simulink subsystem "Plataforma_IGBT"  (R2024b)
settings: Solver=VariableStepAuto  StartTime=0.0  StopTime=10.0  RelTol=1e-3
values from neighbouring files (symbols this model uses):
  R_L = mean(RL)    [backup_0907.m]    (also in controller_0107.m = 0.01; matlabfunction_0207_ukf.m = 0.1)
  Ts = 0.001    [boost_data.mat]    (also in teste_ukf.m = 1e-05; wynda_demo.m)
undefined symbols (not defined in the file or in its folder): f_cutoff, var_HV, var_LV
libraries: fl_lib x18, ee_lib x18, nesl_utility x15
settings Model: Creator=eric  LastModifiedBy=eric

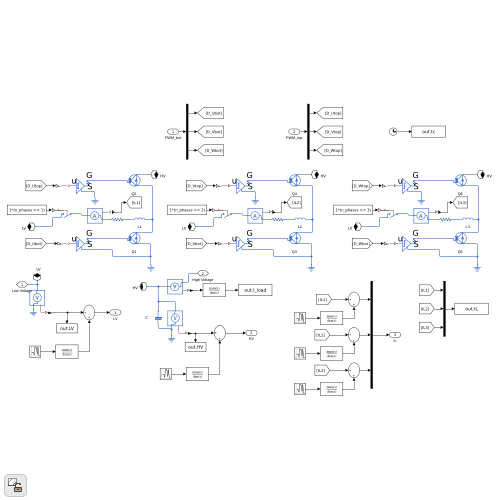
[thumbnail: Simulink's stored preview of the top-level diagram]
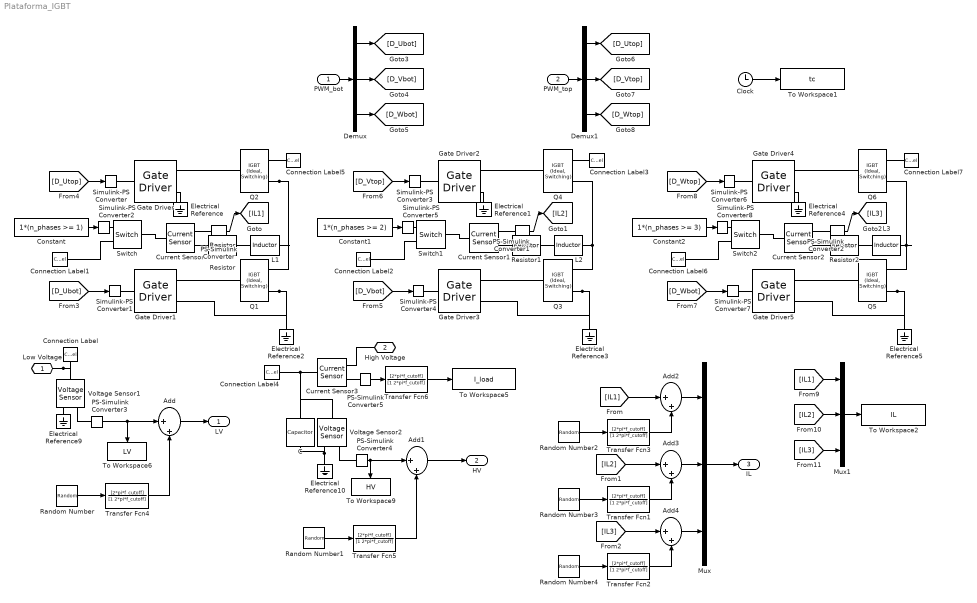
== system Plataforma_IGBT ==
  PWM_bot : Inport
  PWM_top : Inport  Port=2
  Add{,1..4} (5 alike) : Sum  Inputs=|++
  C : fl_lib/Electrical/Electrical Elements/Capacitor  c=C_out mF  r=C_out_esr mOhm  g=0 1/Ohm  i_specify=off  i_priority=None  i=0 A  i_nominal_specify=off  i_nominal_value=1  i_nominal_unit=A  v_specify=on  v_priority=None  v=12 V  v_nominal_specify=off  v_nominal_value=1  v_nominal_unit=V  vc_specify=off  vc_priority=High  vc=0 V  vc_nominal_specify=off  vc_nominal_value=1  vc_nominal_unit=V
  Clock : Clock
      settings: Decimation=decim
  Connection Label{,1..2,6} (4 alike) : ConnectionLabel  Label=LV
  Connection Label{3..5,7} (4 alike) : ConnectionLabel  Label=HV
  Constant : Constant  Value=1*(n_phases >= 1)
  Constant1 : Constant  Value=1*(n_phases >= 2)
  Constant2 : Constant  Value=1*(n_phases >= 3)
  Current Sensor{,1..3} (4 alike) : fl_lib/Electrical/Electrical Sensors/Current Sensor
  Demux : Demux  Outputs=3
  Demux1 : Demux  Outputs=3
  Electrical Reference{,1..5,9..10} (8 alike) : fl_lib/Electrical/Electrical Elements/Electrical Reference
  Gate Driver{,1..5} (6 alike) : ee_lib/Semiconductors & Converters/Gate Driver  port_option=ee.enum.controlport.ps  uHigh=2.0 V  uLow=0.8 V  uHighValue=0.7  uLowValue=0.3  vHigh=15 V  vLow=0 V  tHigh=50 ns  tLow=50 ns  parameterization=ee.enum.semiconductors.gateDriverParam.outputImpedance  rHigh=2 Ohm  rLow=2 Ohm  tRise=20 ns  tFall=20 ns  cLoad=10 nF  t_fault=1 s  ZonTime_specify=off  ZonTime_priority=None  ZonTime=0 s  ZoffTime_specify=off  ZoffTime_priority=None  ZoffTime=0 s
      settings: InternalSimscapePortConfiguration="{\"Bottom\":[],\"Left\":[{\"id\":\"u\",\"label\":\"u\",\"type\":\"input\"}],\"Right\":[{\"id\":\"G\",\"label\":\"G\",\"type\":\"foundation.electrical.electrical\"},{\"id\":\"S\",\"label\":\"S\",\"type\":\"foundation.electrical.electrical\"}],\"Top\":[]}"
  L1 : ee_lib/Passive/Inductor  l=L mH  enable_L_tol=ee.enum.toleranceApplication.applyRand  L_tol=10  tol_distribution=ee.enum.toleranceDistribution.uniform  nSigma=4  r=0 mOhm  g=1e-9 1/Ohm  enable_operating_limits=ee.enum.enable.no  operating_limit_action=ee.enum.passive.reportOpLim.warn  max_working_current=1 A  power_rating=1 W  fault_action=simscape.enum.assert.action.none  t_fault=1 s  i_L_specify=off  i_L_priority=High  i_L=0 A  i_L_nominal_specify=off  i_L_nominal_value=1  i_L_nominal_unit=A
  L2 : ee_lib/Passive/Inductor  l=L mH  enable_L_tol=ee.enum.toleranceApplication.applyRand  L_tol=10  tol_distribution=ee.enum.toleranceDistribution.uniform  nSigma=4  r=0 mOhm  g=1e-9 1/Ohm  enable_operating_limits=ee.enum.enable.no  operating_limit_action=ee.enum.passive.reportOpLim.warn  max_working_current=1 A  power_rating=1 W  fault_action=simscape.enum.assert.action.none  t_fault=1 s  i_L_specify=off  i_L_priority=High  i_L=0 A  i_L_nominal_specify=off  i_L_nominal_value=1  i_L_nominal_unit=A
  L3 : ee_lib/Passive/Inductor  l=L mH  enable_L_tol=ee.enum.toleranceApplication.applyRand  L_tol=10  tol_distribution=ee.enum.toleranceDistribution.uniform  nSigma=4  r=0 mOhm  g=1e-9 1/Ohm  enable_operating_limits=ee.enum.enable.no  operating_limit_action=ee.enum.passive.reportOpLim.warn  max_working_current=1 A  power_rating=1 W  fault_action=simscape.enum.assert.action.none  t_fault=1 s  i_L_specify=off  i_L_priority=High  i_L=0 A  i_L_nominal_specify=off  i_L_nominal_value=1  i_L_nominal_unit=A
  Mux : Mux  Inputs=3
  Mux1 : Mux  Inputs=3
  PS-Simulink Converter{,1..5} (6 alike) : nesl_utility/PS-Simulink Converter  PhysicalDomain=network_engine_domain  SubClassName=ps_output  LeftPortType=input  RightPortType=output  PseudoPeriodic=off  Frequencies=[]  VectorFormat=inherit  Unit=inherit  AffineConversion=off
  Q{1..6} (6 alike) : ee_lib/Semiconductors & Converters/IGBT (Ideal, Switching)  port_option=ee.enum.controlport.elec  Vf=0.8 V  Ron=0.001 Ohm  Goff=1e-5 1/Ohm  Vth=6 V  diode_param=ee.enum.semiconductors.protectionDiode.nodynamics  diode_Vf=0.8 V  diode_Ron=0.001 Ohm  diode_Goff=1e-5 1/Ohm  diode_C=50e-9 F  diode_iRM=-235 A  diode_iF=300 A  diode_idot=-50 A/us  diode_trr_param=ee.enum.converters.diodeReverseParam.trr_factor  diode_trr_factor=3  diode_trr=15 us  diode_Qrr=1500 s*uA  ice_specify=off  ice_priority=None  ice=0 A  ice_nominal_specify=off  ice_nominal_value=1  ice_nominal_unit=A  vce_specify=off  vce_priority=None  vce=0 V  vce_nominal_specify=off  vce_nominal_value=1  vce_nominal_unit=V  vge_specify=off  vge_priority=None  vge=0 V  vge_nominal_specify=off  vge_nominal_value=1  vge_nominal_unit=V  thermal_loss_option=ee.enum.converters.thermalLossOption.constantvalues  Von_data=[0, .1, .6, .8, 1, 1.3, 1.6, 2, 2.4; 0, .1, .7, 1, 1.2, 1.5, 1.9, 2.4, 2.8] V  Tj=[298.15, 398.15] K  Iout_data=[0, .1, 1, 5, 10, 20, 40, 70, 100] A  Eon_data=[0, .0024, .024, .12, .2, .48, 1.04, 2.16, 3.24; 0, .003, .03, .15, .25, .6, 1.3, 2.7, 4.05] * 1e-3 J  Eoff_data=[0, .0007, .0066, .033, .066, .17, .33, .83, 1.5; 0, .001, .01, .05, .1, .25, .5, 1.2, 2.2] * 1e-3 J  Eon_data_3D=[zeros(2, 9, 3)] J  Eoff_data_3D=[zeros(2, 9, 3)] J  Tj_loss=[298.15, 398.15] K  Iout_data_loss=[0, .1, 1, 5, 10, 20, 40, 70, 100] A  tabulateWithVce=false  Vce_loss=[0, 150, 300] V  Eon_scalar=22.86e-3 J  Eoff_scalar=17.14e-3 J  Voff=300 V  Iout_scalar=600 A  useCurrentFromPreviousCycle=false  useVoltageFromPreviousCycle=false  diodeModelType=ee.enum.converters.diodeModelType.pwl  diodeTableType=ee.enum.diode.tableType.IfMat  diode_ReverseIVType=ee.enum.diode.diodeReverseIV.constant  diode_IfMat=[.07, .12, .19, 1.75, 4.24, 7.32, 11.2; .16, .3, .72, 2.14, 4.02, 6.35, 9.12] A  diode_VfMat=[.9, 1.15, 1.25, 1.5, 1.75, 2.17, 2.6, 2.85; .58, .68, .75, 1.1, 1.38, 1.77, 2.27, 2.7] V  diode_TjVec=[25, 125] degC  diode_VfVec=[.5, .7, .9, 1.3, 1.7, 2.1, 2.5] V  diode_IfVec=[.1, .2, .5, 1, 2, 4, 7, 10] A  diode_IrMat=[1e-06, 2e-06, 5e-06, 1e-05, 2.5e-05, 5e-05, .0001; 2e-06, 5e-06, 1e-05, 4e-05, 8e-05, .0002, .0005] A  diode_VrMat=[10, 100, 200, 250, 300, 325, 350; 10, 70, 160, 220, 270, 300, 320] V  diode_VrVec=[10, 20, 40, 50, 70, 80, 100] V  diode_IrVec=[1e-06, 2e-06, 5e-06, 1e-05, 2e-05, 5e-05, .0001] A  diode_Vr=-600 V  diode_Ls=150 nH  diode_Erec=0.03 J  diode_rec_loss_model=ee.enum.diode.reverseRecoveryModel.fixed  diode_ErecVal=0 J  diode_scaleWithIandV=true  diode_ErecMat=zeros(2, 3) J  diode_TjrecVec=[298.15, 398.15] K  diode_IfrecVec=[.1, 1, 10] A  diode_IrecVal=10 A  diode_VrecVal=10 V  diode_tFilter=1 / 1000 / 100 s  separateThermalPortForDiode=false  thermal_network_parameterization=ee.enum.thermalNetworkTopology.external  Rth=[.08, .5] K/W  Rth_Cauer=[.08, .1, .5] K/W  Rth_Foster=[.08, .14, .22, .16] K/W  thermal_mass_parameterization=ee.enum.thermalNetwork.timeconstant  thermal_mass=[.01, .5] J/K  thermal_mass_Cauer=[.01, .1, .5] J/K  thermal_mass_Foster=[.001, .005, .05, .5] J/K  thermal_time_constant=[.001, .2] s  thermal_time_constant_Cauer=[.001, .1, .2] s  thermal_time_constant_Foster=[7e-05, .0007, .01, .08] s  thermal_mass_initial_temperatures=[25, 25] degC  thermal_mass_initial_temperatures_Cauer=[25, 25, 25] degC  junction_thermal_mass=0.01 J/K  Tvec_initial_Foster=[25, 25, 25, 25] degC  RthDiode=[.03, .2] K/W  RthCauerDiode=[.03, .1, .2] K/W  RthFosterDiode=[.03, .2] K/W  thermalMassDiode=[3, 25] J/K  thermalMassCauerDiode=[3, 10, 25] J/K  thermalMassFosterDiode=[33, 50] J/K  thermalTauDiode=[.1, 5] s  thermalTauCauerDiode=[.1, 1, 5] s  thermalTauFosterDiode=[1, 10] s  thermalMassInitTempDiode=[25, 25] degC  thermalMassInitTempCauerDiode=[25, 25, 25] degC  junctionthermalMassDiode=0.1 J/K  TVecInitialFosterDiode=[25, 25, 25, 25] degC  no_thermal_network=0  IGBT_junction_temperature_specify=off  IGBT_junction_temperature_priority=None  IGBT_junction_temperature=25 degC  IGBT_junction_temperature_nominal_specify=off  IGBT_junction_temperature_nominal_value=1  IGBT_junction_temperature_nominal_unit=degC  diode_junction_temperature_specify=off  diode_junction_temperature_priority=None  diode_junction_temperature=25 degC  diode_junction_temperature_nominal_specify=off  diode_junction_temperature_nominal_value=1  diode_junction_temperature_nominal_unit=degC  Qj_specify=off  Qj_priority=None  Qj=0 W  Qj_nominal_specify=off  Qj_nominal_value=1  Qj_nominal_unit=W  accumulatedSwitchingLosses_specify=off  accumulatedSwitchingLosses_priority=None  accumulatedSwitchingLosses=0 J
      settings: InternalSimscapePortConfiguration="{\"Bottom\":[],\"Left\":[{\"id\":\"G_elec\",\"label\":\"\",\"type\":\"foundation.electrical.electrical\"}],\"Right\":[{\"id\":\"C\",\"label\":\"\",\"type\":\"foundation.electrical.electrical\"},{\"id\":\"E\",\"label\":\"\",\"type\":\"foundation.electrical.electrical\"}],\"Top\":[]}"
  Random Number : RandomNumber  Variance=var_LV  SampleTime=Ts
  Random Number{1..4} (4 alike) : RandomNumber  Variance=var_HV  SampleTime=Ts
  Resistor : ee_lib/Passive/Resistor  R=R_L mOhm  enable_R_tol=ee.enum.toleranceApplication.applyRand  R_tol=50  tol_distribution=ee.enum.toleranceDistribution.uniform  nSigma=4  enable_operating_limits=ee.enum.enable.no  operating_limit_action=ee.enum.passive.reportOpLim.warn  power_rating=1 W  max_working_voltage=100 V  noise_mode=ee.enum.sources.noise.Disabled  Tdevice=25 degC  sample_time=1e-3 s  repeatability=ee.enum.ic.repeatability.notRepeatable  user_seed=0  auto_seed=3499211588  fault_action=simscape.enum.assert.action.none  t_fault=1 s  power_derating_T1=70 degC  power_derating_T2=155 degC  operating_temperature_range_vec=[-50, 150] degC  alpha=3.93e-3 1/K  Tmeas=25 degC  thermal_mass=100 J/K  temperature_specify=off  temperature_priority=High  temperature=298.15 K  temperature_nominal_specify=off  temperature_nominal_value=1  temperature_nominal_unit=K
  Resistor1 : ee_lib/Passive/Resistor  R=R_L mOhm  enable_R_tol=ee.enum.toleranceApplication.applyRand  R_tol=50  tol_distribution=ee.enum.toleranceDistribution.uniform  nSigma=4  enable_operating_limits=ee.enum.enable.no  operating_limit_action=ee.enum.passive.reportOpLim.warn  power_rating=1 W  max_working_voltage=100 V  noise_mode=ee.enum.sources.noise.Disabled  Tdevice=25 degC  sample_time=1e-3 s  repeatability=ee.enum.ic.repeatability.notRepeatable  user_seed=0  auto_seed=3890346746  fault_action=simscape.enum.assert.action.none  t_fault=1 s  power_derating_T1=70 degC  power_derating_T2=155 degC  operating_temperature_range_vec=[-50, 150] degC  alpha=3.93e-3 1/K  Tmeas=25 degC  thermal_mass=100 J/K  temperature_specify=off  temperature_priority=High  temperature=298.15 K  temperature_nominal_specify=off  temperature_nominal_value=1  temperature_nominal_unit=K
  Resistor2 : ee_lib/Passive/Resistor  R=R_L mOhm  enable_R_tol=ee.enum.toleranceApplication.applyRand  R_tol=50  tol_distribution=ee.enum.toleranceDistribution.uniform  nSigma=4  enable_operating_limits=ee.enum.enable.no  operating_limit_action=ee.enum.passive.reportOpLim.warn  power_rating=1 W  max_working_voltage=100 V  noise_mode=ee.enum.sources.noise.Disabled  Tdevice=25 degC  sample_time=1e-3 s  repeatability=ee.enum.ic.repeatability.notRepeatable  user_seed=0  auto_seed=545404223  fault_action=simscape.enum.assert.action.none  t_fault=1 s  power_derating_T1=70 degC  power_derating_T2=155 degC  operating_temperature_range_vec=[-50, 150] degC  alpha=3.93e-3 1/K  Tmeas=25 degC  thermal_mass=100 J/K  temperature_specify=off  temperature_priority=High  temperature=298.15 K  temperature_nominal_specify=off  temperature_nominal_value=1  temperature_nominal_unit=K
  Simulink-PS Converter{,1..8} (9 alike) : nesl_utility/Simulink-PS Converter  PhysicalDomain=network_engine_domain  SubClassName=ps_input  LeftPortType=input  RightPortType=output  PseudoPeriodic=off  Frequencies=[]  NoiseDistribution=none  NoiseParameters=[]  Unit=1  AffineConversion=off  FilteringAndDerivatives=provide  SimscapeFilterOrder=1  InputFilterTimeConstant=0.001  UdotUserProvided=0
  Switch : fl_lib/Electrical/Electrical Elements/Switch  R_closed=0.01 mOhm  G_open=1e-8 1/Ohm  Threshold=0.5  i_specify=off  i_priority=None  i=0 A  i_nominal_specify=off  i_nominal_value=1  i_nominal_unit=A  v_specify=off  v_priority=None  v=0 V  v_nominal_specify=off  v_nominal_value=1  v_nominal_unit=V
  Switch1 : fl_lib/Electrical/Electrical Elements/Switch  R_closed=0.01 mOhm  G_open=1e-8 1/Ohm  Threshold=0.5  i_specify=off  i_priority=None  i=0 A  i_nominal_specify=off  i_nominal_value=1  i_nominal_unit=A  v_specify=off  v_priority=None  v=0 V  v_nominal_specify=off  v_nominal_value=1  v_nominal_unit=V
  Switch2 : fl_lib/Electrical/Electrical Elements/Switch  R_closed=0.01 mOhm  G_open=1e-8 1/Ohm  Threshold=0.5  i_specify=off  i_priority=None  i=0 A  i_nominal_specify=off  i_nominal_value=1  i_nominal_unit=A  v_specify=off  v_priority=None  v=0 V  v_nominal_specify=off  v_nominal_value=1  v_nominal_unit=V
  To Workspace1 : ToWorkspace  VariableName=tc  SampleTime=-1
      settings: Decimation=decim  Save2DSignal=2-D array (concatenate along first dimension)
  To Workspace2 : ToWorkspace  VariableName=IL  SampleTime=-1
      settings: Decimation=decim  Save2DSignal=2-D array (concatenate along first dimension)
  To Workspace5 : ToWorkspace  VariableName=I_load  SampleTime=-1
      settings: Decimation=decim  Save2DSignal=2-D array (concatenate along first dimension)
  To Workspace6 : ToWorkspace  VariableName=LV  SampleTime=-1
      settings: Decimation=decim  Save2DSignal=2-D array (concatenate along first dimension)
  To Workspace9 : ToWorkspace  VariableName=HV  SampleTime=-1
      settings: Decimation=decim  Save2DSignal=2-D array (concatenate along first dimension)
  Transfer Fcn{1..6} (6 alike) : TransferFcn  Numerator=[2*pi*f_cutoff]  Denominator=[1 2*pi*f_cutoff]  ContinuousStateAttributes='LV'
  Voltage Sensor1 : fl_lib/Electrical/Electrical Sensors/Voltage Sensor
  Voltage Sensor2 : fl_lib/Electrical/Electrical Sensors/Voltage Sensor
  Low Voltage : PMIOPort  Side=Left
  High Voltage : PMIOPort  Port=2  Side=Left
  LV : Outport
  HV : Outport  Port=2
  IL : Outport  Port=3
  wires:
  [D_Utop] -> Simulink-PS Converter/1
  [IL1] -> Add2/1
  Mux/1 -> IL/1
  PWM_bot/1 -> Demux/1
  Demux/1 -> [D_Ubot]
  Demux/2 -> [D_Vbot]
  Demux/3 -> [D_Wbot]
  Demux1/1 -> [D_Utop]
  Demux1/2 -> [D_Vtop]
  PWM_top/1 -> Demux1/1
  Demux1/3 -> [D_Wtop]
  Constant/1 -> Simulink-PS Converter2/1
  [D_Ubot] -> Simulink-PS Converter1/1
  PS-Simulink Converter/1 -> [IL1]
  [D_Vbot] -> Simulink-PS Converter4/1
  PS-Simulink Converter1/1 -> [IL2]
  [D_Vtop] -> Simulink-PS Converter3/1
  Constant1/1 -> Simulink-PS Converter5/1
  [D_Wbot] -> Simulink-PS Converter7/1
  PS-Simulink Converter2/1 -> [IL3]
  [D_Wtop] -> Simulink-PS Converter6/1
  Constant2/1 -> Simulink-PS Converter8/1
  Add2/1 -> Mux/1
  Add3/1 -> Mux/2
  Add4/1 -> Mux/3
  Add1/1 -> HV/1
  PS-Simulink Converter3/1 -> To Workspace6/1, Add/1
  PS-Simulink Converter4/1 -> To Workspace9/1, Add1/1
  [IL1] -> Mux1/1
  [IL2] -> Mux1/2
  [IL3] -> Mux1/3
  Mux1/1 -> To Workspace2/1
  Random Number/1 -> Transfer Fcn4/1
  Transfer Fcn4/1 -> Add/2
  Add/1 -> LV/1
  Random Number1/1 -> Transfer Fcn5/1
  Transfer Fcn5/1 -> Add1/2
  Transfer Fcn3/1 -> Add2/2
  Random Number2/1 -> Transfer Fcn3/1
  Random Number3/1 -> Transfer Fcn1/1
  Transfer Fcn1/1 -> Add3/2
  Random Number4/1 -> Transfer Fcn2/1
  Transfer Fcn2/1 -> Add4/2
  [IL2] -> Add3/1
  [IL3] -> Add4/1
  Clock/1 -> To Workspace1/1
  PS-Simulink Converter5/1 -> Transfer Fcn6/1
  Transfer Fcn6/1 -> To Workspace5/1
  connections:
  Q2/RConn2 -- L1/LConn1 -- Q1/RConn1
  Low Voltage/RConn1 -- Connection Label/LConn1 -- Voltage Sensor1/LConn1
  Electrical Reference10/LConn1 -- C/RConn1 -- Voltage Sensor2/RConn2
  Connection Label4/LConn1 -- C/LConn1 -- Voltage Sensor2/LConn1 -- Current Sensor3/LConn1
  Q1/RConn2 -- Gate Driver1/RConn2 -- Electrical Reference2/LConn1
  Q3/RConn1 -- Q4/RConn2 -- L2/LConn1
  Q3/RConn2 -- Gate Driver3/RConn2 -- Electrical Reference3/LConn1
  Q5/RConn1 -- L3/LConn1 -- Q6/RConn2
  Q5/RConn2 -- Gate Driver5/RConn2 -- Electrical Reference5/LConn1
  Switch/LConn1 -- Current Sensor/LConn1
  Gate Driver/RConn1 -- Q2/LConn1
  Simulink-PS Converter/RConn1 -- Gate Driver/LConn1
  Electrical Reference/LConn1 -- Gate Driver/RConn2
  Gate Driver1/RConn1 -- Q1/LConn1
  Current Sensor/RConn2 -- Resistor/LConn1
  PS-Simulink Converter/LConn1 -- Current Sensor/RConn1
  PS-Simulink Converter3/LConn1 -- Voltage Sensor1/RConn1
  Connection Label5/LConn1 -- Q2/RConn1
  Electrical Reference9/LConn1 -- Voltage Sensor1/RConn2
  PS-Simulink Converter4/LConn1 -- Voltage Sensor2/RConn1
  Switch/RConn2 -- Connection Label1/LConn1
  PS-Simulink Converter5/LConn1 -- Current Sensor3/RConn1
  Simulink-PS Converter2/RConn1 -- Switch/RConn1
  High Voltage/RConn1 -- Current Sensor3/RConn2
  Gate Driver1/LConn1 -- Simulink-PS Converter1/RConn1
  Simulink-PS Converter5/RConn1 -- Switch1/RConn1
  Gate Driver3/RConn1 -- Q3/LConn1
  Gate Driver3/LConn1 -- Simulink-PS Converter4/RConn1
  Switch1/RConn2 -- Connection Label2/LConn1
  Current Sensor1/RConn2 -- Resistor1/LConn1
  Gate Driver2/RConn1 -- Q4/LConn1
  Connection Label3/LConn1 -- Q4/RConn1
  Electrical Reference1/LConn1 -- Gate Driver2/RConn2
  PS-Simulink Converter1/LConn1 -- Current Sensor1/RConn1
  Switch1/LConn1 -- Current Sensor1/LConn1
  Simulink-PS Converter3/RConn1 -- Gate Driver2/LConn1
  Simulink-PS Converter8/RConn1 -- Switch2/RConn1
  Gate Driver5/RConn1 -- Q5/LConn1
  Gate Driver5/LConn1 -- Simulink-PS Converter7/RConn1
  Switch2/RConn2 -- Connection Label6/LConn1
  Resistor2/LConn1 -- Current Sensor2/RConn2
  Gate Driver4/RConn1 -- Q6/LConn1
  Connection Label7/LConn1 -- Q6/RConn1
  Electrical Reference4/LConn1 -- Gate Driver4/RConn2
  PS-Simulink Converter2/LConn1 -- Current Sensor2/RConn1
  Switch2/LConn1 -- Current Sensor2/LConn1
  Simulink-PS Converter6/RConn1 -- Gate Driver4/LConn1
  Resistor/RConn1 -- L1/RConn1
  Resistor1/RConn1 -- L2/RConn1
  L3/RConn1 -- Resistor2/RConn1
